simulink model "softMBD_old"  (R2025b)
settings: Solver=FixedStepAuto  StartTime=0.0  StopTime=10  FixedStep=0.005  RelTol=1e-3
values from neighbouring files (symbols this model uses):
  FPV_mass = 0.8    [Soft.m]
  g = 9.81    [Soft.m]
  ks = 0    [Soft.m]
  p_0 = 1013.25    [Soft.m]
  Q2Ts = forcetomotors()    [Soft.m]    (also in forcetomotors.m = inv(Ts2Q))
  takeOffDuration = 2    [Soft.m]
  Ts = 0.005    [Soft.m]
undefined symbols (not defined in the file or in its folder): DiscIntNeverNeededParam, kd_pq, kd_pr, kd_y, ki_pq, ki_pr, ki_t, ki_y, kp_pq, kp_pr, kp_y, pInitialization
libraries: simulink x35, discretizing x11, slpidlib x2, shared6dof x1, dynamicsLibrary x1, aerolibasang x1, aerolibnav x1
(part 9 of 20)

== system softMBD_old/FCS/Controller/position_controller/PID Controller2/Ideal P Gain ==
  In1 : Inport  SampleTime=SampleTime
  P Gain : Inport  Port=2  SampleTime=SampleTime
  External Parameters : Subsystem  VariantControl=ExternalParameters
  Internal Parameters : Subsystem  VariantControl=InternalParameters
  Passthrough : Subsystem  VariantControl=Disabled
  Out1 : Outport  SampleTime=SampleTime

== system softMBD_old/FCS/Controller/position_controller/PID Controller2/Ideal P Gain Fdbk ==
  In1 : Inport  SampleTime=SampleTime
  P Gain : Inport  Port=2  SampleTime=SampleTime
  Disabled : Subsystem  VariantControl=Disabled
  External Parameters : Subsystem  VariantControl=ExternalParameters
  Internal Parameters : Subsystem  VariantControl=InternalParameters
  Passthrough : Subsystem  VariantControl=Passthrough
  Out1 : Outport  SampleTime=SampleTime

== system softMBD_old/FCS/Controller/position_controller/PID Controller2/Integrator ==
  U : Inport  SampleTime=SampleTime
  I0in : Inport  Port=2  SampleTime=SampleTime
  Reset : Inport  Port=3  SampleTime=SampleTime
  Continuous : Subsystem  VariantControl=Continuous
  Disabled : Subsystem  VariantControl=Disabled
  Discrete : Subsystem  VariantControl=Discrete
  state : Outport  SampleTime=SampleTime
  out : Outport  Port=2  SampleTime=SampleTime

== system softMBD_old/FCS/Controller/position_controller/PID Controller2/Integrator ICs ==
  I0 : Inport  SampleTime=SampleTime
  Disabled : Subsystem  VariantControl=Disabled
  External IC : Subsystem  VariantControl=ExternalICs
  Internal IC : Subsystem  VariantControl=InternalICs
  Out1 : Outport  SampleTime=SampleTime

== system softMBD_old/FCS/Controller/position_controller/PID Controller2/N Copy ==
  N Gain : Inport  SampleTime=SampleTime
  Disabled : Subsystem  VariantControl=Disabled
  Disabled wSignal Specification : Subsystem  VariantControl=Disabled_SignalSpec
  External Parameters : Subsystem  VariantControl=ExternalParameters
  Internal Parameters : Subsystem  VariantControl=InternalParameters
  Out1 : Outport  SampleTime=SampleTime

== system softMBD_old/FCS/Controller/position_controller/PID Controller2/N Gain ==
  U : Inport  SampleTime=SampleTime
  N Gain : Inport  Port=2  SampleTime=SampleTime
  Disabled : Subsystem  VariantControl=Disabled
  External Parameters : Subsystem  VariantControl=ExternalParameters
  Internal Parameters : Subsystem  VariantControl=InternalParameters
  Passthrough : Subsystem  VariantControl=Passthrough
  Out1 : Outport  SampleTime=SampleTime

== system softMBD_old/FCS/Controller/position_controller/PID Controller2/P Copy ==
  P Gain : Inport  SampleTime=SampleTime
  Disabled : Subsystem  VariantControl=Disabled
  External Parameters Ideal : Subsystem  VariantControl=ExternalParamsIdeal
  Internal Parameters Ideal : Subsystem  VariantControl=InternalParamsIdeal
  Out1 : Outport  SampleTime=SampleTime

== system softMBD_old/FCS/Controller/position_controller/PID Controller2/PID Compensator Formula ==

== system softMBD_old/FCS/Controller/position_controller/PID Controller2/Parallel P Gain ==
  err : Inport  SampleTime=SampleTime
  P Gain : Inport  Port=2  SampleTime=SampleTime
  Disabled : Subsystem  VariantControl=Disabled
  External Parameters : Subsystem  VariantControl=ExternalParameters
  Internal Parameters : Subsystem  VariantControl=InternalParameters
  Passthrough : Subsystem  VariantControl=Passthrough
  Out1 : Outport  SampleTime=SampleTime

== system softMBD_old/FCS/Controller/position_controller/PID Controller2/Reset Signal ==
  Reset : Inport  SampleTime=SampleTime
  Disabled : Subsystem  VariantControl=Disabled
  External Reset : Subsystem  VariantControl=ExternalReset
  Out1 : Outport  SampleTime=SampleTime

== system softMBD_old/FCS/Controller/position_controller/PID Controller2/Saturation ==
  In1 : Inport  SampleTime=SampleTime
  Upper Limit : Inport  Port=2  SampleTime=SampleTime
  Lower Limit : Inport  Port=3  SampleTime=SampleTime
  Enabled : Subsystem  VariantControl=Enabled
  External : Subsystem  VariantControl=External
  Passthrough : Subsystem  VariantControl=Disabled
  Out1 : Outport  SampleTime=SampleTime

== system softMBD_old/FCS/Controller/position_controller/PID Controller2/Saturation Fdbk ==
  In1 : Inport  SampleTime=SampleTime
  Upper Limit : Inport  Port=2  SampleTime=SampleTime
  Lower Limit : Inport  Port=3  SampleTime=SampleTime
  Disabled : Subsystem  VariantControl=Disabled
  Enabled : Subsystem  VariantControl=Enabled
  External : Subsystem  VariantControl=External
  Passthrough : Subsystem  VariantControl=Passthrough
  Out1 : Outport  SampleTime=SampleTime

== system softMBD_old/FCS/Controller/position_controller/PID Controller2/Sum ==
  P : Inport  SampleTime=SampleTime
  I : Inport  Port=2  SampleTime=SampleTime
  D : Inport  Port=3  SampleTime=SampleTime
  Passthrough_I : Subsystem  VariantControl=Passthrough_I
  Passthrough_P : Subsystem  VariantControl=Passthrough_P
  Sum_PD : Subsystem  VariantControl=Sum_PD
  Sum_PI : Subsystem  VariantControl=Sum_PI
  Sum_PID : Subsystem  VariantControl=Sum_PID
  Out1 : Outport  SampleTime=SampleTime

== system softMBD_old/FCS/Controller/position_controller/PID Controller2/Sum Fdbk ==
  fromP : Inport  SampleTime=SampleTime
  fromState : Inport  Port=2  SampleTime=SampleTime
  fromD : Inport  Port=3  SampleTime=SampleTime
  Disabled : Subsystem  VariantControl=Disabled
  Enabled : Subsystem  VariantControl=Enabled
  Passthrough : Subsystem  VariantControl=Passthrough
  Out1 : Outport  SampleTime=SampleTime

== system softMBD_old/FCS/Controller/position_controller/PID Controller2/Tracking Mode ==
  uout : Inport  SampleTime=SampleTime
  TR : Inport  Port=2  SampleTime=SampleTime
  Disabled : Subsystem  VariantControl=Disabled
  Enabled : Subsystem  VariantControl=Enabled
  Out1 : Outport  SampleTime=SampleTime

== system softMBD_old/FCS/Controller/position_controller/PID Controller2/Tracking Mode Sum ==
  fromIgain : Inport  SampleTime=SampleTime
  fromTR : Inport  Port=2  SampleTime=SampleTime
  Passthrough : Subsystem  VariantControl=Passthrough
  Tracking Mode : Subsystem  VariantControl=TrackingMode
  preInt : Outport

== system softMBD_old/FCS/Controller/position_controller/PID Controller2/Tsamp - Integral ==
  U : Inport  SampleTime=SampleTime
  Ts : Inport  Port=2  SampleTime=SampleTime
  Disabled : Subsystem  VariantControl=Disabled
  External Ts : Subsystem  VariantControl=ExternalTs
  Passthrough : Subsystem  VariantControl=Passthrough
  TsSignalSpecification : Subsystem  VariantControl=Disabled_SignalSpec
  Out1 : Outport  SampleTime=SampleTime

== system softMBD_old/FCS/Controller/position_controller/PID Controller2/Tsamp - Ngain ==
  U : Inport  SampleTime=SampleTime
  Ts : Inport  Port=2  SampleTime=SampleTime
  External Ts : Subsystem  VariantControl=ExternalTs
  Passthrough : Subsystem  VariantControl=Passthrough
  Out1 : Outport  SampleTime=SampleTime

== system softMBD_old/FCS/Controller/position_controller/PID Controller2/postSat Signal ==
  feedback : Inport  SampleTime=SampleTime
  forward : Inport  Port=2  SampleTime=SampleTime
  Feedback_Path : Subsystem  VariantControl=Feedback
  Forward_Path : Subsystem  VariantControl=Forward
  Out1 : Outport  SampleTime=SampleTime

== system softMBD_old/FCS/Controller/position_controller/PID Controller2/preInt Signal ==
  preInt : Inport  SampleTime=SampleTime
  extAW : Inport  Port=2  SampleTime=SampleTime
  External PreInt : Subsystem  VariantControl=ExternalPreInt
  Internal PreInt : Subsystem  VariantControl=InternalPreInt
  Out1 : Outport  SampleTime=SampleTime

== system softMBD_old/FCS/Controller/position_controller/PID Controller2/preSat Signal ==
  feedback : Inport  SampleTime=SampleTime
  forward : Inport  Port=2  SampleTime=SampleTime
  Feedback_Path : Subsystem  VariantControl=Feedback
  Forward_Path : Subsystem  VariantControl=Forward
  Out1 : Outport  SampleTime=SampleTime

== system softMBD_old/FCS/Controller/position_controller/PID Controller3/Anti-windup ==
  preSat : Inport  SampleTime=SampleTime
  postSat : Inport  Port=2  SampleTime=SampleTime
  P : Inport  Port=3  SampleTime=SampleTime
  preInt : Inport  Port=4  SampleTime=SampleTime
  Upper Limit : Inport  Port=5  SampleTime=SampleTime
  Lower Limit : Inport  Port=6  SampleTime=SampleTime
  Back Calculation : Subsystem  VariantControl=BackCalculation
  Cont. Clamping Ideal : Subsystem  VariantControl=ContClampingIdeal
  Cont. Clamping Parallel : Subsystem  VariantControl=ContClampingParallel
  Disabled : Subsystem  VariantControl=Disabled
  Disc. Clamping Ideal : Subsystem  VariantControl=DiscClampingIdeal
  Disc. Clamping Parallel : Subsystem  VariantControl=DiscClampingParallel
  Passthrough : Subsystem  VariantControl=Passthrough
  Out1 : Outport  SampleTime=SampleTime

== system softMBD_old/FCS/Controller/position_controller/PID Controller3/D Gain ==
  err : Inport  SampleTime=SampleTime
  D Gain : Inport  Port=2  SampleTime=SampleTime
  Disabled : Subsystem  VariantControl=Disabled
  External Parameters : Subsystem  VariantControl=ExternalParameters
  Internal Parameters : Subsystem  VariantControl=InternalParameters
  Out1 : Outport  SampleTime=SampleTime

== system softMBD_old/FCS/Controller/position_controller/PID Controller3/External Derivative ==
  err : Inport  SampleTime=SampleTime
  ydot : Inport  Port=2  SampleTime=SampleTime
  Disabled : Subsystem  VariantControl=Disabled
  Error : Subsystem  VariantControl=ErrorSignal
  External Ydot : Subsystem  VariantControl=ExternalYdot
  Out1 : Outport  SampleTime=SampleTime

== system softMBD_old/FCS/Controller/position_controller/PID Controller3/Filter ==
  Reset : Inport  SampleTime=SampleTime
  U : Inport  Port=2  SampleTime=SampleTime
  N : Inport  Port=3  SampleTime=SampleTime
  D0in : Inport  Port=4  SampleTime=SampleTime
  Nout : Inport  Port=5  SampleTime=SampleTime
  Ts : Inport  Port=6  SampleTime=SampleTime
  Cont. Filter : Subsystem  VariantControl=ContFilter
  Cont. Filter Only : Subsystem  VariantControl=ContFilterOnly
  Differentiator : Subsystem  VariantControl=Differentiator
  Disabled : Subsystem  VariantControl=Disabled
  Disc. Backward Euler Filter : Subsystem  VariantControl=BackwardEulerFilter
  Disc. Backward Euler Filter Only : Subsystem  VariantControl=BackwardEulerFilterOnly
  Disc. Forward Euler Filter : Subsystem  VariantControl=ForwardEulerFilter
  Disc. Forward Euler Filter Only : Subsystem  VariantControl=ForwardEulerFilterOnly
  Disc. Trapezoidal Filter : Subsystem  VariantControl=TrapezoidalFilter
  Disc. Trapezoidal Filter Only : Subsystem  VariantControl=TrapezoidalFilterOnly
  Passthrough : Subsystem  VariantControl=Passthrough
  Y : Outport  SampleTime=SampleTime

== system softMBD_old/FCS/Controller/position_controller/PID Controller3/Filter ICs ==
  D0 : Inport  SampleTime=SampleTime
  Disabled : Subsystem  VariantControl=Disabled
  External IC : Subsystem  VariantControl=ExternalICs
  Internal IC - Differentiator : Subsystem  VariantControl=InternalICsDifferentiator
  Internal IC - Filter : Subsystem  VariantControl=InternalICsFilter
  Out1 : Outport  SampleTime=SampleTime

== system softMBD_old/FCS/Controller/position_controller/PID Controller3/I Gain ==
  err : Inport  SampleTime=SampleTime
  I Gain : Inport  Port=2  SampleTime=SampleTime
  Disabled : Subsystem  VariantControl=Disabled
  External Parameters : Subsystem  VariantControl=ExternalParameters
  Internal Parameters : Subsystem  VariantControl=InternalParameters
  Out1 : Outport  SampleTime=SampleTime

== system softMBD_old/FCS/Controller/position_controller/PID Controller3/Ideal P Gain ==
  In1 : Inport  SampleTime=SampleTime
  P Gain : Inport  Port=2  SampleTime=SampleTime
  External Parameters : Subsystem  VariantControl=ExternalParameters
  Internal Parameters : Subsystem  VariantControl=InternalParameters
  Passthrough : Subsystem  VariantControl=Disabled
  Out1 : Outport  SampleTime=SampleTime

== system softMBD_old/FCS/Controller/position_controller/PID Controller3/Ideal P Gain Fdbk ==
  In1 : Inport  SampleTime=SampleTime
  P Gain : Inport  Port=2  SampleTime=SampleTime
  Disabled : Subsystem  VariantControl=Disabled
  External Parameters : Subsystem  VariantControl=ExternalParameters
  Internal Parameters : Subsystem  VariantControl=InternalParameters
  Passthrough : Subsystem  VariantControl=Passthrough
  Out1 : Outport  SampleTime=SampleTime

== system softMBD_old/FCS/Controller/position_controller/PID Controller3/Integrator ==
  U : Inport  SampleTime=SampleTime
  I0in : Inport  Port=2  SampleTime=SampleTime
  Reset : Inport  Port=3  SampleTime=SampleTime
  Continuous : Subsystem  VariantControl=Continuous
  Disabled : Subsystem  VariantControl=Disabled
  Discrete : Subsystem  VariantControl=Discrete
  state : Outport  SampleTime=SampleTime
  out : Outport  Port=2  SampleTime=SampleTime

== system softMBD_old/FCS/Controller/position_controller/PID Controller3/Integrator ICs ==
  I0 : Inport  SampleTime=SampleTime
  Disabled : Subsystem  VariantControl=Disabled
  External IC : Subsystem  VariantControl=ExternalICs
  Internal IC : Subsystem  VariantControl=InternalICs
  Out1 : Outport  SampleTime=SampleTime

== system softMBD_old/FCS/Controller/position_controller/PID Controller3/N Copy ==
  N Gain : Inport  SampleTime=SampleTime
  Disabled : Subsystem  VariantControl=Disabled
  Disabled wSignal Specification : Subsystem  VariantControl=Disabled_SignalSpec
  External Parameters : Subsystem  VariantControl=ExternalParameters
  Internal Parameters : Subsystem  VariantControl=InternalParameters
  Out1 : Outport  SampleTime=SampleTime

== system softMBD_old/FCS/Controller/position_controller/PID Controller3/N Gain ==
  U : Inport  SampleTime=SampleTime
  N Gain : Inport  Port=2  SampleTime=SampleTime
  Disabled : Subsystem  VariantControl=Disabled
  External Parameters : Subsystem  VariantControl=ExternalParameters
  Internal Parameters : Subsystem  VariantControl=InternalParameters
  Passthrough : Subsystem  VariantControl=Passthrough
  Out1 : Outport  SampleTime=SampleTime

== system softMBD_old/FCS/Controller/position_controller/PID Controller3/P Copy ==
  P Gain : Inport  SampleTime=SampleTime
  Disabled : Subsystem  VariantControl=Disabled
  External Parameters Ideal : Subsystem  VariantControl=ExternalParamsIdeal
  Internal Parameters Ideal : Subsystem  VariantControl=InternalParamsIdeal
  Out1 : Outport  SampleTime=SampleTime

== system softMBD_old/FCS/Controller/position_controller/PID Controller3/PID Compensator Formula ==

== system softMBD_old/FCS/Controller/position_controller/PID Controller3/Parallel P Gain ==
  err : Inport  SampleTime=SampleTime
  P Gain : Inport  Port=2  SampleTime=SampleTime
  Disabled : Subsystem  VariantControl=Disabled
  External Parameters : Subsystem  VariantControl=ExternalParameters
  Internal Parameters : Subsystem  VariantControl=InternalParameters
  Passthrough : Subsystem  VariantControl=Passthrough
  Out1 : Outport  SampleTime=SampleTime

== system softMBD_old/FCS/Controller/position_controller/PID Controller3/Reset Signal ==
  Reset : Inport  SampleTime=SampleTime
  Disabled : Subsystem  VariantControl=Disabled
  External Reset : Subsystem  VariantControl=ExternalReset
  Out1 : Outport  SampleTime=SampleTime

== system softMBD_old/FCS/Controller/position_controller/PID Controller3/Saturation ==
  In1 : Inport  SampleTime=SampleTime
  Upper Limit : Inport  Port=2  SampleTime=SampleTime
  Lower Limit : Inport  Port=3  SampleTime=SampleTime
  Enabled : Subsystem  VariantControl=Enabled
  External : Subsystem  VariantControl=External
  Passthrough : Subsystem  VariantControl=Disabled
  Out1 : Outport  SampleTime=SampleTime

== system softMBD_old/FCS/Controller/position_controller/PID Controller3/Saturation Fdbk ==
  In1 : Inport  SampleTime=SampleTime
  Upper Limit : Inport  Port=2  SampleTime=SampleTime
  Lower Limit : Inport  Port=3  SampleTime=SampleTime
  Disabled : Subsystem  VariantControl=Disabled
  Enabled : Subsystem  VariantControl=Enabled
  External : Subsystem  VariantControl=External
  Passthrough : Subsystem  VariantControl=Passthrough
  Out1 : Outport  SampleTime=SampleTime

== system softMBD_old/FCS/Controller/position_controller/PID Controller3/Sum ==
  P : Inport  SampleTime=SampleTime
  I : Inport  Port=2  SampleTime=SampleTime
  D : Inport  Port=3  SampleTime=SampleTime
  Passthrough_I : Subsystem  VariantControl=Passthrough_I
  Passthrough_P : Subsystem  VariantControl=Passthrough_P
  Sum_PD : Subsystem  VariantControl=Sum_PD
  Sum_PI : Subsystem  VariantControl=Sum_PI
  Sum_PID : Subsystem  VariantControl=Sum_PID
  Out1 : Outport  SampleTime=SampleTime

== system softMBD_old/FCS/Controller/position_controller/PID Controller3/Sum Fdbk ==
  fromP : Inport  SampleTime=SampleTime
  fromState : Inport  Port=2  SampleTime=SampleTime
  fromD : Inport  Port=3  SampleTime=SampleTime
  Disabled : Subsystem  VariantControl=Disabled
  Enabled : Subsystem  VariantControl=Enabled
  Passthrough : Subsystem  VariantControl=Passthrough
  Out1 : Outport  SampleTime=SampleTime

== system softMBD_old/FCS/Controller/position_controller/PID Controller3/Tracking Mode ==
  uout : Inport  SampleTime=SampleTime
  TR : Inport  Port=2  SampleTime=SampleTime
  Disabled : Subsystem  VariantControl=Disabled
  Enabled : Subsystem  VariantControl=Enabled
  Out1 : Outport  SampleTime=SampleTime

== system softMBD_old/FCS/Controller/position_controller/PID Controller3/Tracking Mode Sum ==
  fromIgain : Inport  SampleTime=SampleTime
  fromTR : Inport  Port=2  SampleTime=SampleTime
  Passthrough : Subsystem  VariantControl=Passthrough
  Tracking Mode : Subsystem  VariantControl=TrackingMode
  preInt : Outport

== system softMBD_old/FCS/Controller/position_controller/PID Controller3/Tsamp - Integral ==
  U : Inport  SampleTime=SampleTime
  Ts : Inport  Port=2  SampleTime=SampleTime
  Disabled : Subsystem  VariantControl=Disabled
  External Ts : Subsystem  VariantControl=ExternalTs
  Passthrough : Subsystem  VariantControl=Passthrough
  TsSignalSpecification : Subsystem  VariantControl=Disabled_SignalSpec
  Out1 : Outport  SampleTime=SampleTime

== system softMBD_old/FCS/Controller/position_controller/PID Controller3/Tsamp - Ngain ==
  U : Inport  SampleTime=SampleTime
  Ts : Inport  Port=2  SampleTime=SampleTime
  External Ts : Subsystem  VariantControl=ExternalTs
  Passthrough : Subsystem  VariantControl=Passthrough
  Out1 : Outport  SampleTime=SampleTime

== system softMBD_old/FCS/Controller/position_controller/PID Controller3/postSat Signal ==
  feedback : Inport  SampleTime=SampleTime
  forward : Inport  Port=2  SampleTime=SampleTime
  Feedback_Path : Subsystem  VariantControl=Feedback
  Forward_Path : Subsystem  VariantControl=Forward
  Out1 : Outport  SampleTime=SampleTime

== system softMBD_old/FCS/Controller/position_controller/PID Controller3/preInt Signal ==
  preInt : Inport  SampleTime=SampleTime
  extAW : Inport  Port=2  SampleTime=SampleTime
  External PreInt : Subsystem  VariantControl=ExternalPreInt
  Internal PreInt : Subsystem  VariantControl=InternalPreInt
  Out1 : Outport  SampleTime=SampleTime

== system softMBD_old/FCS/Controller/position_controller/PID Controller3/preSat Signal ==
  feedback : Inport  SampleTime=SampleTime
  forward : Inport  Port=2  SampleTime=SampleTime
  Feedback_Path : Subsystem  VariantControl=Feedback
  Forward_Path : Subsystem  VariantControl=Forward
  Out1 : Outport  SampleTime=SampleTime

== system softMBD_old/FCS/Controller/roll_pitch_controller/PID Controller/Anti-windup ==
  preSat : Inport  SampleTime=SampleTime
  postSat : Inport  Port=2  SampleTime=SampleTime
  P : Inport  Port=3  SampleTime=SampleTime
  preInt : Inport  Port=4  SampleTime=SampleTime
  Upper Limit : Inport  Port=5  SampleTime=SampleTime
  Lower Limit : Inport  Port=6  SampleTime=SampleTime
  Back Calculation : Subsystem  VariantControl=BackCalculation
  Cont. Clamping Ideal : Subsystem  VariantControl=ContClampingIdeal
  Cont. Clamping Parallel : Subsystem  VariantControl=ContClampingParallel
  Disabled : Subsystem  VariantControl=Disabled
  Disc. Clamping Ideal : Subsystem  VariantControl=DiscClampingIdeal
  Disc. Clamping Parallel : Subsystem  VariantControl=DiscClampingParallel
  Passthrough : Subsystem  VariantControl=Passthrough
  Out1 : Outport  SampleTime=SampleTime

== system softMBD_old/FCS/Controller/roll_pitch_controller/PID Controller/D Gain ==
  err : Inport  SampleTime=SampleTime
  D Gain : Inport  Port=2  SampleTime=SampleTime
  Disabled : Subsystem  VariantControl=Disabled
  External Parameters : Subsystem  VariantControl=ExternalParameters
  Internal Parameters : Subsystem  VariantControl=InternalParameters
  Out1 : Outport  SampleTime=SampleTime

== system softMBD_old/FCS/Controller/roll_pitch_controller/PID Controller/External Derivative ==
  err : Inport  SampleTime=SampleTime
  ydot : Inport  Port=2  SampleTime=SampleTime
  Disabled : Subsystem  VariantControl=Disabled
  Error : Subsystem  VariantControl=ErrorSignal
  External Ydot : Subsystem  VariantControl=ExternalYdot
  Out1 : Outport  SampleTime=SampleTime

== system softMBD_old/FCS/Controller/roll_pitch_controller/PID Controller/Filter ==
  Reset : Inport  SampleTime=SampleTime
  U : Inport  Port=2  SampleTime=SampleTime
  N : Inport  Port=3  SampleTime=SampleTime
  D0in : Inport  Port=4  SampleTime=SampleTime
  Nout : Inport  Port=5  SampleTime=SampleTime
  Ts : Inport  Port=6  SampleTime=SampleTime
  Cont. Filter : Subsystem  VariantControl=ContFilter
  Cont. Filter Only : Subsystem  VariantControl=ContFilterOnly
  Differentiator : Subsystem  VariantControl=Differentiator
  Disabled : Subsystem  VariantControl=Disabled
  Disc. Backward Euler Filter : Subsystem  VariantControl=BackwardEulerFilter
  Disc. Backward Euler Filter Only : Subsystem  VariantControl=BackwardEulerFilterOnly
  Disc. Forward Euler Filter : Subsystem  VariantControl=ForwardEulerFilter
  Disc. Forward Euler Filter Only : Subsystem  VariantControl=ForwardEulerFilterOnly
  Disc. Trapezoidal Filter : Subsystem  VariantControl=TrapezoidalFilter
  Disc. Trapezoidal Filter Only : Subsystem  VariantControl=TrapezoidalFilterOnly
  Passthrough : Subsystem  VariantControl=Passthrough
  Y : Outport  SampleTime=SampleTime

== system softMBD_old/FCS/Controller/roll_pitch_controller/PID Controller/Filter ICs ==
  D0 : Inport  SampleTime=SampleTime
  Disabled : Subsystem  VariantControl=Disabled
  External IC : Subsystem  VariantControl=ExternalICs
  Internal IC - Differentiator : Subsystem  VariantControl=InternalICsDifferentiator
  Internal IC - Filter : Subsystem  VariantControl=InternalICsFilter
  Out1 : Outport  SampleTime=SampleTime

== system softMBD_old/FCS/Controller/roll_pitch_controller/PID Controller/I Gain ==
  err : Inport  SampleTime=SampleTime
  I Gain : Inport  Port=2  SampleTime=SampleTime
  Disabled : Subsystem  VariantControl=Disabled
  External Parameters : Subsystem  VariantControl=ExternalParameters
  Internal Parameters : Subsystem  VariantControl=InternalParameters
  Out1 : Outport  SampleTime=SampleTime

== system softMBD_old/FCS/Controller/roll_pitch_controller/PID Controller/Ideal P Gain ==
  In1 : Inport  SampleTime=SampleTime
  P Gain : Inport  Port=2  SampleTime=SampleTime
  External Parameters : Subsystem  VariantControl=ExternalParameters
  Internal Parameters : Subsystem  VariantControl=InternalParameters
  Passthrough : Subsystem  VariantControl=Disabled
  Out1 : Outport  SampleTime=SampleTime

== system softMBD_old/FCS/Controller/roll_pitch_controller/PID Controller/Ideal P Gain Fdbk ==
  In1 : Inport  SampleTime=SampleTime
  P Gain : Inport  Port=2  SampleTime=SampleTime
  Disabled : Subsystem  VariantControl=Disabled
  External Parameters : Subsystem  VariantControl=ExternalParameters
  Internal Parameters : Subsystem  VariantControl=InternalParameters
  Passthrough : Subsystem  VariantControl=Passthrough
  Out1 : Outport  SampleTime=SampleTime

== system softMBD_old/FCS/Controller/roll_pitch_controller/PID Controller/Integrator ==
  U : Inport  SampleTime=SampleTime
  I0in : Inport  Port=2  SampleTime=SampleTime
  Reset : Inport  Port=3  SampleTime=SampleTime
  Continuous : Subsystem  VariantControl=Continuous
  Disabled : Subsystem  VariantControl=Disabled
  Discrete : Subsystem  VariantControl=Discrete
  state : Outport  SampleTime=SampleTime
  out : Outport  Port=2  SampleTime=SampleTime

== system softMBD_old/FCS/Controller/roll_pitch_controller/PID Controller/Integrator ICs ==
  I0 : Inport  SampleTime=SampleTime
  Disabled : Subsystem  VariantControl=Disabled
  External IC : Subsystem  VariantControl=ExternalICs
  Internal IC : Subsystem  VariantControl=InternalICs
  Out1 : Outport  SampleTime=SampleTime

== system softMBD_old/FCS/Controller/roll_pitch_controller/PID Controller/N Copy ==
  N Gain : Inport  SampleTime=SampleTime
  Disabled : Subsystem  VariantControl=Disabled
  Disabled wSignal Specification : Subsystem  VariantControl=Disabled_SignalSpec
  External Parameters : Subsystem  VariantControl=ExternalParameters
  Internal Parameters : Subsystem  VariantControl=InternalParameters
  Out1 : Outport  SampleTime=SampleTime

== system softMBD_old/FCS/Controller/roll_pitch_controller/PID Controller/N Gain ==
  U : Inport  SampleTime=SampleTime
  N Gain : Inport  Port=2  SampleTime=SampleTime
  Disabled : Subsystem  VariantControl=Disabled
  External Parameters : Subsystem  VariantControl=ExternalParameters
  Internal Parameters : Subsystem  VariantControl=InternalParameters
  Passthrough : Subsystem  VariantControl=Passthrough
  Out1 : Outport  SampleTime=SampleTime

== system softMBD_old/FCS/Controller/roll_pitch_controller/PID Controller/P Copy ==
  P Gain : Inport  SampleTime=SampleTime
  Disabled : Subsystem  VariantControl=Disabled
  External Parameters Ideal : Subsystem  VariantControl=ExternalParamsIdeal
  Internal Parameters Ideal : Subsystem  VariantControl=InternalParamsIdeal
  Out1 : Outport  SampleTime=SampleTime

== system softMBD_old/FCS/Controller/roll_pitch_controller/PID Controller/PID Compensator Formula ==

== system softMBD_old/FCS/Controller/roll_pitch_controller/PID Controller/Parallel P Gain ==
  err : Inport  SampleTime=SampleTime
  P Gain : Inport  Port=2  SampleTime=SampleTime
  Disabled : Subsystem  VariantControl=Disabled
  External Parameters : Subsystem  VariantControl=ExternalParameters
  Internal Parameters : Subsystem  VariantControl=InternalParameters
  Passthrough : Subsystem  VariantControl=Passthrough
  Out1 : Outport  SampleTime=SampleTime

== system softMBD_old/FCS/Controller/roll_pitch_controller/PID Controller/Reset Signal ==
  Reset : Inport  SampleTime=SampleTime
  Disabled : Subsystem  VariantControl=Disabled
  External Reset : Subsystem  VariantControl=ExternalReset
  Out1 : Outport  SampleTime=SampleTime

== system softMBD_old/FCS/Controller/roll_pitch_controller/PID Controller/Saturation ==
  In1 : Inport  SampleTime=SampleTime
  Upper Limit : Inport  Port=2  SampleTime=SampleTime
  Lower Limit : Inport  Port=3  SampleTime=SampleTime
  Enabled : Subsystem  VariantControl=Enabled
  External : Subsystem  VariantControl=External
  Passthrough : Subsystem  VariantControl=Disabled
  Out1 : Outport  SampleTime=SampleTime

== system softMBD_old/FCS/Controller/roll_pitch_controller/PID Controller/Saturation Fdbk ==
  In1 : Inport  SampleTime=SampleTime
  Upper Limit : Inport  Port=2  SampleTime=SampleTime
  Lower Limit : Inport  Port=3  SampleTime=SampleTime
  Disabled : Subsystem  VariantControl=Disabled
  Enabled : Subsystem  VariantControl=Enabled
  External : Subsystem  VariantControl=External
  Passthrough : Subsystem  VariantControl=Passthrough
  Out1 : Outport  SampleTime=SampleTime

== system softMBD_old/FCS/Controller/roll_pitch_controller/PID Controller/Sum ==
  P : Inport  SampleTime=SampleTime
  I : Inport  Port=2  SampleTime=SampleTime
  D : Inport  Port=3  SampleTime=SampleTime
  Passthrough_I : Subsystem  VariantControl=Passthrough_I
  Passthrough_P : Subsystem  VariantControl=Passthrough_P
  Sum_PD : Subsystem  VariantControl=Sum_PD
  Sum_PI : Subsystem  VariantControl=Sum_PI
  Sum_PID : Subsystem  VariantControl=Sum_PID
  Out1 : Outport  SampleTime=SampleTime

== system softMBD_old/FCS/Controller/roll_pitch_controller/PID Controller/Sum Fdbk ==
  fromP : Inport  SampleTime=SampleTime
  fromState : Inport  Port=2  SampleTime=SampleTime
  fromD : Inport  Port=3  SampleTime=SampleTime
  Disabled : Subsystem  VariantControl=Disabled
  Enabled : Subsystem  VariantControl=Enabled
  Passthrough : Subsystem  VariantControl=Passthrough
  Out1 : Outport  SampleTime=SampleTime

== system softMBD_old/FCS/Controller/roll_pitch_controller/PID Controller/Tracking Mode ==
  uout : Inport  SampleTime=SampleTime
  TR : Inport  Port=2  SampleTime=SampleTime
  Disabled : Subsystem  VariantControl=Disabled
  Enabled : Subsystem  VariantControl=Enabled
  Out1 : Outport  SampleTime=SampleTime

== system softMBD_old/FCS/Controller/roll_pitch_controller/PID Controller/Tracking Mode Sum ==
  fromIgain : Inport  SampleTime=SampleTime
  fromTR : Inport  Port=2  SampleTime=SampleTime
  Passthrough : Subsystem  VariantControl=Passthrough
  Tracking Mode : Subsystem  VariantControl=TrackingMode
  preInt : Outport

== system softMBD_old/FCS/Controller/roll_pitch_controller/PID Controller/Tsamp - Integral ==
  U : Inport  SampleTime=SampleTime
  Ts : Inport  Port=2  SampleTime=SampleTime
  Disabled : Subsystem  VariantControl=Disabled
  External Ts : Subsystem  VariantControl=ExternalTs
  Passthrough : Subsystem  VariantControl=Passthrough
  TsSignalSpecification : Subsystem  VariantControl=Disabled_SignalSpec
  Out1 : Outport  SampleTime=SampleTime

== system softMBD_old/FCS/Controller/roll_pitch_controller/PID Controller/Tsamp - Ngain ==
  U : Inport  SampleTime=SampleTime
  Ts : Inport  Port=2  SampleTime=SampleTime
  External Ts : Subsystem  VariantControl=ExternalTs
  Passthrough : Subsystem  VariantControl=Passthrough
  Out1 : Outport  SampleTime=SampleTime

== system softMBD_old/FCS/Controller/roll_pitch_controller/PID Controller/postSat Signal ==
  feedback : Inport  SampleTime=SampleTime
  forward : Inport  Port=2  SampleTime=SampleTime
  Feedback_Path : Subsystem  VariantControl=Feedback
  Forward_Path : Subsystem  VariantControl=Forward
  Out1 : Outport  SampleTime=SampleTime

== system softMBD_old/FCS/Controller/roll_pitch_controller/PID Controller/preInt Signal ==
  preInt : Inport  SampleTime=SampleTime
  extAW : Inport  Port=2  SampleTime=SampleTime
  External PreInt : Subsystem  VariantControl=ExternalPreInt
  Internal PreInt : Subsystem  VariantControl=InternalPreInt
  Out1 : Outport  SampleTime=SampleTime

== system softMBD_old/FCS/Controller/roll_pitch_controller/PID Controller/preSat Signal ==
  feedback : Inport  SampleTime=SampleTime
  forward : Inport  Port=2  SampleTime=SampleTime
  Feedback_Path : Subsystem  VariantControl=Feedback
  Forward_Path : Subsystem  VariantControl=Forward
  Out1 : Outport  SampleTime=SampleTime

== system softMBD_old/FCS/filters/Subsystem/x,y,z,dy,dy,dz/x.y.dx.dy ==
  ax : Inport
  ay : Inport  Port=2
  Integrator1 : DiscreteIntegrator  SampleTime=0.005  ICPrevOutput=DiscIntNeverNeededParam  ICPrevScaledInput=DiscIntNeverNeededParam  mask(DiscretizedDiscreteIntegrator){}
      mask init:
      | %zoh
  Integrator2 : DiscreteIntegrator  SampleTime=0.005  ICPrevOutput=DiscIntNeverNeededParam  ICPrevScaledInput=DiscIntNeverNeededParam  mask(DiscretizedDiscreteIntegrator){}
      mask init:
      | %zoh
  Integrator4 : DiscreteIntegrator  SampleTime=0.005  ICPrevOutput=DiscIntNeverNeededParam  ICPrevScaledInput=DiscIntNeverNeededParam  mask(DiscretizedDiscreteIntegrator){}
      mask init:
      | %zoh
  Integrator5 : DiscreteIntegrator  SampleTime=0.005  ICPrevOutput=DiscIntNeverNeededParam  ICPrevScaledInput=DiscIntNeverNeededParam  mask(DiscretizedDiscreteIntegrator){}
      mask init:
      | %zoh
  dx : Outport
  dy : Outport  Port=2
  x : Outport  Port=3
  y : Outport  Port=4
  wires:
  ay/1 -> Integrator2/1
  ax/1 -> Integrator4/1
  Integrator4/1 -> Integrator1/1, dx/1
  Integrator1/1 -> x/1
  Integrator2/1 -> Integrator5/1, dy/1
  Integrator5/1 -> y/1

== system softMBD_old/FCS/filters/Subsystem/x,y,z,dy,dy,dz/z,dz ==
  az : Inport
  pressure_f : Inport  Port=2
  Add : Sum  Inputs=+-
  Constant : Constant  Value=p_0  OutDataTypeStr=single
  Demux : Demux  Outputs=2
  Gain : Gain  Gain=1/12.01  OutDataTypeStr=single
  Kalman Filter1 : Subsystem  AncestorBlock=cstblocks/State Estimation/Kalman Filter  mask(ctrlKalmanFilter){TimeDomain=Discrete-Time, UseCurrentEstimator=on, ModelSource=Individual A, B, C, D matrices, ModelSourceVariable=ss(0.95,1,1,0,1), A=[1 Ts;0 1], B=[0.5*Ts^2; Ts], C=[1 0], D=0, NumberOfStates=1, NumberOfInputs=1, NumberOfOutputs=1, InitialEstimateSource=Dialog, X0=0, P0=10, UseK=off, UseGH=off, NumberOfProcessNoiseInputs=1, G=1, TimeInvariantG=on, H=0, TimeInvariantH=on, Q=0.001, TimeInvariantQ=on, R=0.1, TimeInvariantR=on, N=0, TimeInvariantN=on, AddInputPort=on, AddEnablePort=off, ExternalReset=None, OutputEstimatedY=off, OutputP=off, Ts=Ts}
      mask prompts: TimeDomain "Controllib:blocks:maskPromptKFTimeDomain"; UseCurrentEstimator "Controllib:blocks:maskPromptKFUseCurrentMeasurement"; ModelSource "Controllib:blocks:maskPromptKFModelSource"; ModelSourceVariable "Controllib:blocks:maskPromptKFModelSourceVariable"; A "Controllib:blocks:maskPromptKFA"; B "Controllib:blocks:maskPromptKFB"; C "Controllib:blocks:maskPromptKFC"; D "Controllib:blocks:maskPromptKFD"; NumberOfStates "Controllib:blocks:maskPromptKFNumberOfStates"; NumberOfInputs "Controllib:blocks:maskPromptKFNumberOfInputs"; NumberOfOutputs "Controllib:blocks:maskPromptKFNumberOfOutputs"; InitialEstimateSource "Controllib:blocks:maskPromptKFSource"; X0 "Controllib:blocks:maskPromptKFX0DT"; P0 "Controllib:blocks:maskPromptKFP0DT"; UseK "Controllib:blocks:maskPromptKFUseK"; UseGH "Controllib:blocks:maskPromptKFUseGH"; NumberOfProcessNoiseInputs "Controllib:blocks:maskPromptKFNumberOfProcessNoiseInputs"; G "Controllib:blocks:maskPromptKFG"; TimeInvariantG "Controllib:blocks:maskPromptKFTimeInvariantG"; H "Controllib:blocks:maskPromptKFH"; TimeInvariantH "Controllib:blocks:maskPromptKFTimeInvariantH"; Q "Controllib:blocks:maskPromptKFQ"; TimeInvariantQ "Controllib:blocks:maskPromptKFTimeInvariantQ"; R "Controllib:blocks:maskPromptKFR"; TimeInvariantR "Controllib:blocks:maskPromptKFTimeInvariantR"; N "Controllib:blocks:maskPromptKFN"; TimeInvariantN "Controllib:blocks:maskPromptKFTimeInvariantN"; AddInputPort "Controllib:blocks:maskPromptKFAddInputPort"; AddEnablePort "Controllib:blocks:maskPromptKFAddEnablePort"; ExternalReset "Simulink:blkprm_prompts:DelayBlkExternalReset"; OutputEstimatedY "Controllib:blocks:maskPromptKFOutputEstimatedY"; OutputP "Controllib:blocks:maskPromptKFOutputPZ"; Ts "Controllib:blocks:maskPromptKFTs"
      mask help: Controllib:blocks:maskPromptKFDescription
      mask init: same as softMBD_old/FCS/filters/Subsystem1/pitch_kalman/Kalman Filter1
      settings: LibrarySourceBlock=cstblocks/State Estimation/Kalman Filter
      mask Help: eval('controllib.internal.blocks.kalmanfilter.launchDocPage()')
      mask TypeOptions TimeDomain: Controllib:blocks:maskPromptKFTimeDomainDT | Controllib:blocks:maskPromptKFTimeDomainCT
      mask Callback TimeDomain: controllib.internal.blocks.kalmanfilter.dialogCallbacks(gcbh(),'comboBoxTimeDomain');
      mask Callback UseCurrentEstimator: controllib.internal.blocks.kalmanfilter.dialogCallbacks(gcbh(),'checkBoxUseCurrentEstimator');
      mask TypeOptions ModelSource: Controllib:blocks:maskPromptKFModelSourceLTIObject | Controllib:blocks:maskPromptKFModelSourceMatrices | Controllib:blocks:maskPromptKFSourceInport
      mask Callback ModelSource: controllib.internal.blocks.kalmanfilter.dialogCallbacks(gcbh(),'comboBoxModelSource');
      mask Callback ModelSourceVariable: controllib.internal.blocks.kalmanfilter.dialogCallbacks(gcbh(),'editBoxModelSourceVariable')
      mask TypeOptions InitialEstimateSource: Controllib:blocks:maskPromptKFSourceDialog | Controllib:blocks:maskPromptKFSourceInport
      mask Callback InitialEstimateSource: controllib.internal.blocks.kalmanfilter.dialogCallbacks(gcbh(),'comboBoxInitialEstimateSource');
      mask Callback UseK: controllib.internal.blocks.kalmanfilter.dialogCallbacks(gcbh(),'checkBoxUseK');
      mask Callback UseGH: controllib.internal.blocks.kalmanfilter.dialogCallbacks(gcbh(),'checkBoxUseGH');
      mask Callback TimeInvariantG: controllib.internal.blocks.kalmanfilter.dialogCallbacks(gcbh(),'checkBoxTimeInvariantGH');
      mask Callback TimeInvariantH: controllib.internal.blocks.kalmanfilter.dialogCallbacks(gcbh(),'checkBoxTimeInvariantGH');
      mask Callback TimeInvariantQ: controllib.internal.blocks.kalmanfilter.dialogCallbacks(gcbh(),'checkBoxTimeInvariantQRN');
      mask Callback TimeInvariantR: controllib.internal.blocks.kalmanfilter.dialogCallbacks(gcbh(),'checkBoxTimeInvariantQRN');
      mask Callback TimeInvariantN: controllib.internal.blocks.kalmanfilter.dialogCallbacks(gcbh(),'checkBoxTimeInvariantQRN');
      mask Callback AddInputPort: controllib.internal.blocks.kalmanfilter.dialogCallbacks(gcbh(),'checkBoxAddInputPort');
      mask TypeOptions ExternalReset: MemoryX/ExternalReset
      mask Callback OutputP: controllib.internal.blocks.kalmanfilter.dialogCallbacks(gcbh(),'checkBoxOutputP');
      mask DialogControl DescGroupVar Prompt: Controllib:blocks:maskPromptKFTitle
      mask DialogControl FilterSettingsContainer Prompt: Controllib:blocks:maskPromptKFContainerFilterSettings
      mask DialogControl TimeDomain Prompt: Time domain:
      mask DialogControl UseCurrentEstimator Prompt: Use the current measurement y[n] to improve xhat[n]
      mask DialogControl ModelParameterContainer Prompt: Controllib:blocks:maskPromptKFTabModelParameters
      mask DialogControl SystemModelContainer Prompt: Controllib:blocks:maskPromptKFContainerSystemModel
      mask DialogControl ModelSource Prompt: Model source:
      mask DialogControl ModelSourceVariable Prompt: Variable:
      mask DialogControl A Prompt: A:
      mask DialogControl B Prompt: B:
      mask DialogControl C Prompt: C:
      mask DialogControl D Prompt: D:
      mask DialogControl NumberOfStates Prompt: Number of states:
      mask DialogControl NumberOfInputs Prompt: Number of inputs:
      mask DialogControl NumberOfOutputs Prompt: Number of outputs:
      mask DialogControl InitialEstimatesContainer Prompt: Controllib:blocks:maskPromptKFContainerInitialEstimates
      mask DialogControl InitialEstimateSource Prompt: Source:
      mask DialogControl X0 Prompt: Initial states x[0]:
      mask DialogControl P0 Prompt: State estimation error covariance P[0]
      mask DialogControl NoiseCharacteristicsContainer Prompt: Controllib:blocks:maskPromptKFContainerNoiseCharacteristics
      mask DialogControl UseK Prompt: Use the Kalman Gain K from the model variable
      mask DialogControl UseGH Prompt: Use G and H matrices (default G=I and H=0)
      mask DialogControl NumberOfProcessNoiseInputs Prompt: Number of process noise inputs:
      mask DialogControl G Prompt: G:
      mask DialogControl TimeInvariantG Prompt: Time-invariant G
      mask DialogControl H Prompt: H:
      mask DialogControl TimeInvariantH Prompt: Time-invariant H
      mask DialogControl Q Prompt: Q:
      mask DialogControl TimeInvariantQ Prompt: Time-invariant Q
      mask DialogControl R Prompt: R:
      mask DialogControl TimeInvariantR Prompt: Time-invariant R
      mask DialogControl N Prompt: N:
      mask DialogControl TimeInvariantN Prompt: Time-invariant N
      mask DialogControl OptionsContainer Prompt: Controllib:blocks:maskPromptKFTabOptions
      mask DialogControl AdditionalInportsContainer Prompt: Controllib:blocks:maskPromptKFContainerAdditionalInports
      mask DialogControl AddInputPort Prompt: Add input port u
      mask DialogControl AddEnablePort Prompt: Add input port Enable to control measurement updates
      mask DialogControl ExternalReset Prompt: External reset:
      mask DialogControl AdditionalOutportsContainer Prompt: Controllib:blocks:maskPromptKFContainerAdditionalOutports
      mask DialogControl OutputEstimatedY Prompt: Output estimated model output y
      mask DialogControl OutputP Prompt: Output state estimation error covariance Z
      mask DialogControl Ts Prompt: Sample time (-1 for inherited):
  Rate Transition : RateTransition  OutPortSampleTime=Ts
  Rate Transition1 : RateTransition  OutPortSampleTime=Ts
  z : Outport
  dz : Outport  Port=2
  wires:
  Demux/1 -> z/1
  pressure_f/1 -> Add/2
  Constant/1 -> Add/1
  Add/1 -> Gain/1
  Gain/1 -> Rate Transition1/1
  Kalman Filter1/1(xhat) -> Demux/1
  Demux/2 -> dz/1
  Rate Transition/1 -> Kalman Filter1/1(u)
  az/1 -> Rate Transition/1
  Rate Transition1/1 -> Kalman Filter1/2(y)
